simulink model "engine_control"  (R2024a)
settings: Solver=ode4  StartTime=0.0  StopTime=10.0  FixedStep=1e-6  RelTol=1e-3
settings Model: Creator=18283  LastModifiedBy=18283
settings OptimizationCC: DefaultParameterBehavior=Inlined  EnhancedBackFolding=on  PassReuseOutputArgsAs=Individual arguments  ZeroExternalMemoryAtStartup=off  ZeroInternalMemoryAtStartup=off  OptimizeBlockOrder=speed  DifferentSizesBufferReuse=on  OptimizationCustomize=off  EfficientTunableParamExpr=on
settings DebuggingCC: ParameterTunabilityLossMsg=error
settings SFSimCC: MATLABDynamicMemAlloc=off
settings RTWCC: Description=Embedded Coder  SystemTargetFile=ert.tlc  TemplateMakefile=ert_default_tmf
settings CodeAppCC: ForceParamTrailComments=on  IgnoreCustomStorageClasses=off  OperatorAnnotations=on  SimulinkDataObjDesc=on  SFDataObjDesc=on  InsertBlockDesc=on
settings ERTTargetCC: TargetLangStandard=C99 (ISO)  GenerateSampleERTMain=on  InlinedParameterPlacement=NonHierarchical  ERTCustomFileTemplate=example_file_process.tlc

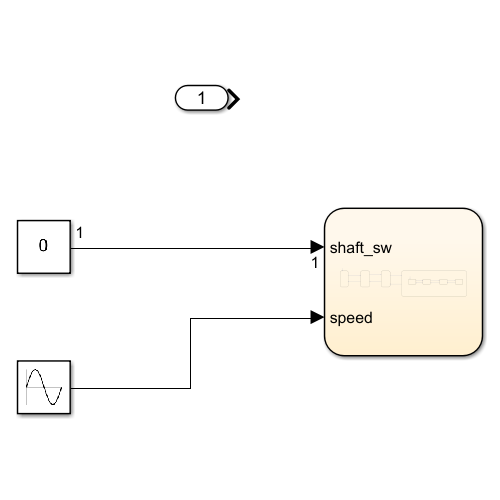
[thumbnail: Simulink's stored preview of the top-level diagram]
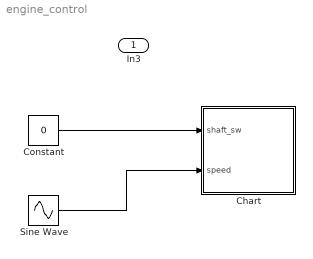
== system engine_control ==
  In3 : Inport
  Chart : Stateflow chart  TreatAsAtomicUnit=on
  Constant : Constant  Value=0
  Sine Wave : Sin  Amplitude=100  SampleTime=0
  wires:
  Constant/1 -> Chart/1(shaft_sw)
  Sine Wave/1 -> Chart/2(speed)

== stateflow chart engine_control/Chart ==
  state P
  state R
  state N
  state D
    state D1
    state D2
    state D3
    state D4
    (default) -> D1
    D3 -> D4 [order 1] : [speed>60]
    D1 -> D2 : [speed>20]
    D2 -> D3 [order 1] : [speed>40]
    D4 -> D3 : [speed<55]
    D3 -> D2 [order 2] : [speed<35]
    D2 -> D1 [order 2] : [speed<15]
  (default) -> P
  R -> N [order 1] : [shift_sw==NN]
  P -> R : [shift_sw==RR]
  N -> D [order 1] : [shift_sw==DD]
  R -> P [order 2] : [shift_sw==PP]
  N -> R [order 2] : [shift_sw==RR]
  D -> N : [shift_sw==NN]
  data: shaft_sw input; speed input
